simulink model "single_phase_full_bridge_inverter"  (R2021a)
settings: Solver=ode23tb  StartTime=0.0  StopTime=2*t  MaxStep=1e-4  RelTol=1e-3
values from neighbouring files (symbols this model uses):
  Ac = 1    [Inverter_parameters.m]
  Ar = ma*Ac    (= 0.5)    [Inverter_parameters.m]
  fc1 = mf1*f    (= 1000)    [Inverter_parameters.m]
  fc2 = mf2*f    (= 1150)    [Inverter_parameters.m]
  fr = 2*pi*f    (= 314.159265359)    [Inverter_parameters.m]
  L = X/(2*pi*f)    (= 0.0999493042617)    [Inverter_parameters.m]
  R = 100    [Inverter_parameters.m]
  Vin = 780    [Inverter_parameters.m]
libraries: spsRMSLib x5, spsIGBTDiodeLib x4, simulink x4, spsCurrentMeasurementLib x2, spsSeriesRLCBranchLib x1, spsVoltageMeasurementLib x1, spsDCVoltageSourceLib x1, spspowerguiLib x1
settings Model: Creator=HossamAladdin  LastModifiedBy=HossamAladdin
settings DataIOCC: ReturnWorkspaceOutputs=off

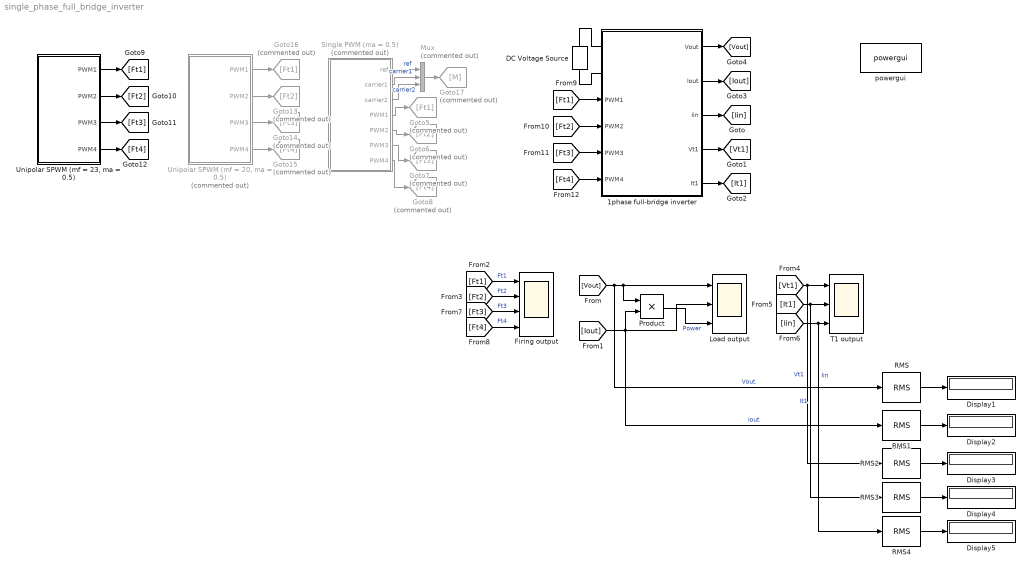
== system single_phase_full_bridge_inverter ==
  1phase full-bridge inverter : Subsystem
      settings: PortSchema="{\"entries\":[{\"content\":{\"sides\":[{\"content\":{\"connectorIds\":[\"LConn1\",\"LConn2\",\"In1\",\"In2\",\"In3\",\"In4\"]},\"type\":\"ConnectorPlacement.EquallySpacedRectSide\",\"uuid\":\"f4e4df3f-ffe1-4ba5-a3cb-8d734668f50c\"},{\"content\":{\"connectorIds\":[\"Out1\",\"Out2\",\"Out3\",\"Out4\",\"Out5\"],\"side\":\"RIGHT\"},\"type\":\"ConnectorPlacement.EquallySpacedRectSide\",\"uuid\":\"90fcdfa8-dce7-4e84-a242-f7f3ace87075\"},{\"content\":{\"connectorIds\":[],\"side\":\"TOP\"},\"type\":\"ConnectorPlacement.EquallySpacedRectSide\",\"uuid\":\"6c6a0c5d-cde1-4235-902c-253094bb6e2c\"}]},\"type\":\"ConnectorPlacement.EquallySpacedConnector\",\"uuid\":\"22214fd6-21aa-42b2-81ed-e947f83e4bbd\"}],\"packageUris\":[\"http://schema.mathworks.com/mf0/Connector/R2020b\"],\"version\":\"1.0\"}"
  DC Voltage Source : spsDCVoltageSourceLib/DC Voltage Source  Amplitude=Vin  Measurements=None
  Display{1..5} (5 alike) : Display
  Firing output : Scope  NumInputPorts=4
  Goto13 : Goto  Commented=on  GotoTag=Ft2
  Goto14 : Goto  Commented=on  GotoTag=Ft3
  Goto15 : Goto  Commented=on  GotoTag=Ft4
  Goto16 : Goto  Commented=on  GotoTag=Ft1
  Goto17 : Goto  Commented=on  GotoTag=M
  Goto5 : Goto  Commented=on  GotoTag=Ft1
  Goto6 : Goto  Commented=on  GotoTag=Ft2
  Goto7 : Goto  Commented=on  GotoTag=Ft3
  Goto8 : Goto  Commented=on  GotoTag=Ft4
  Load output : Scope  NumInputPorts=3
  Mux : Mux  Commented=on  Inputs=3
  Product : Product
  RMS{,1..4} (5 alike) : spsRMSLib/RMS  TrueRMS=on  Freq=50  RMSInit=0  Ts=0
  Single PWM (ma = 0.5) : Subsystem  Commented=on
  T1 output : Scope  NumInputPorts=3
  "Unipolar SPWM (mf = 20, ma = 0.5)" : Subsystem  Commented=on
  "Unipolar SPWM (mf = 23, ma = 0.5)" : Subsystem
  powergui : spspowerguiLib/powergui  Priority=1  SimulationMode=Discrete  SampleTime=1e-6  frequency=60  Iterations=50  frequencyindice=0  Pbase=100e6  ErrMax=1e-4  UnitsV=kV  UnitsW=MW  buscounter=0  FunctionMessages=off  echomessages=off  EnableUseOfTLC=off  CurrentSourceSwitches=off  DisableSnubberDevices=off  DisableRonSwitches=off  DisableVfSwitches=off  DisplayEquations=off  AutomaticDiscreteSolvers=off  SolverType=Tustin/Backward Euler (TBE)  Interpol=off  ExternalGateDelay=off  methode=off  Ts=100  x0status=blocks  SPID=on  SwTol=0  HookPort=off  NonlinearTolerance=1e-4  nMaxIteration=100  ContinueOnMaxIteration=off  RestoreLinks=warning  ResistiveCurrentMeasurement=off  Frange=[0:2:500]  Ylog=off  Xlog=on  ShowGrid=off  save=off  variable=ZData  structure=0  ZoomFFT=off  StartTime=0.0  cycles=1  DisplayStyle=1  fundamental=60  FreqAxis=off  MaxFrequency=1000  frequencyindicesteady=1  RmsSteady=1  display=off
  wires:
  1phase full-bridge inverter/5(It1) -> [It1]
  1phase full-bridge inverter/4(Vt1) -> [Vt1]
  1phase full-bridge inverter/2(Iout) -> [Iout]
  [Vt1] -> T1 output/1, RMS2/1  "Vt1"
  1phase full-bridge inverter/3(Iin) -> [Iin]
  1phase full-bridge inverter/1(Vout) -> [Vout]
  [Vout] -> RMS/1, Load output/1, Product/1  "Vout"
  [Ft2] -> Firing output/2  "Ft2"
  [Ft1] -> Firing output/1  "Ft1"
  [It1] -> T1 output/2, RMS3/1  "It1"
  [Iin] -> RMS4/1, T1 output/3  "Iin"
  [Iout] -> RMS1/1, Product/2, Load output/2  "Iout"
  Product/1 -> Load output/3  "Power"
  Single PWM (ma = 0.5)/4(PWM1) -> Goto5/1
  Single PWM (ma = 0.5)/5(PWM2) -> Goto6/1
  "Unipolar SPWM (mf = 23, ma = 0.5)"/4(PWM4) -> [Ft4]
  "Unipolar SPWM (mf = 23, ma = 0.5)"/1(PWM1) -> [Ft1]
  "Unipolar SPWM (mf = 20, ma = 0.5)"/1(PWM1) -> Goto16/1
  "Unipolar SPWM (mf = 20, ma = 0.5)"/4(PWM4) -> Goto15/1
  [Ft3] -> Firing output/3  "Ft3"
  [Ft4] -> Firing output/4  "Ft4"
  "Unipolar SPWM (mf = 20, ma = 0.5)"/2(PWM2) -> Goto13/1
  "Unipolar SPWM (mf = 20, ma = 0.5)"/3(PWM3) -> Goto14/1
  Single PWM (ma = 0.5)/7(PWM4) -> Goto8/1
  Single PWM (ma = 0.5)/6(PWM3) -> Goto7/1
  "Unipolar SPWM (mf = 23, ma = 0.5)"/2(PWM2) -> [Ft2]
  "Unipolar SPWM (mf = 23, ma = 0.5)"/3(PWM3) -> [Ft3]
  [Ft1] -> 1phase full-bridge inverter/1(PWM1)
  [Ft2] -> 1phase full-bridge inverter/2(PWM2)
  [Ft3] -> 1phase full-bridge inverter/3(PWM3)
  [Ft4] -> 1phase full-bridge inverter/4(PWM4)
  Single PWM (ma = 0.5)/1(ref) -> Mux/1  "ref"
  Single PWM (ma = 0.5)/2(carrier1) -> Mux/2  "carrier1"
  Single PWM (ma = 0.5)/3(carrier2) -> Mux/3  "carrier2"
  Mux/1 -> Goto17/1
  RMS4/1 -> Display5/1
  RMS1/1 -> Display2/1
  RMS3/1 -> Display4/1
  RMS2/1 -> Display3/1
  RMS/1 -> Display1/1
  connections:
  1phase full-bridge inverter/LConn1 -- DC Voltage Source/RConn1
  1phase full-bridge inverter/LConn2 -- DC Voltage Source/LConn1

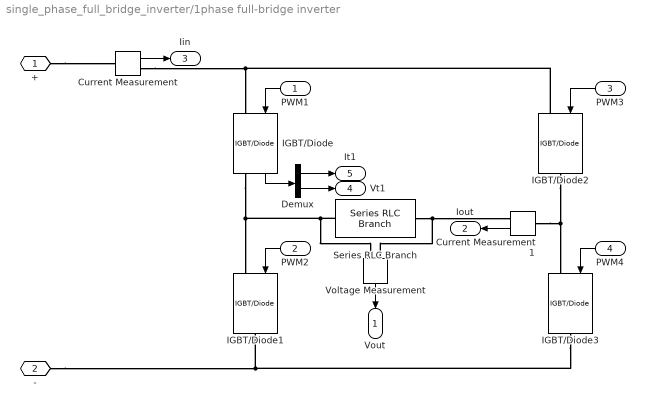
== system single_phase_full_bridge_inverter/1phase full-bridge inverter ==
  PWM1 : Inport
  PWM2 : Inport  Port=2
  PWM3 : Inport  Port=3
  PWM4 : Inport  Port=4
  Current Measurement : spsCurrentMeasurementLib/Current Measurement  PhasorSimulation=off  OutputType=Complex  PSBequivalent=0
  Current Measurement1 : spsCurrentMeasurementLib/Current Measurement  PhasorSimulation=off  OutputType=Complex  PSBequivalent=0
  Demux : Demux  Outputs=2
  IGBT/Diode : spsIGBTDiodeLib/IGBT//Diode  Ron=1e-3  Rs=1e5  Cs=inf  Measurements=on
  IGBT/Diode1 : spsIGBTDiodeLib/IGBT//Diode  Ron=1e-3  Rs=1e5  Cs=inf  Measurements=off
  IGBT/Diode2 : spsIGBTDiodeLib/IGBT//Diode  Ron=1e-3  Rs=1e5  Cs=inf  Measurements=off
  IGBT/Diode3 : spsIGBTDiodeLib/IGBT//Diode  Ron=1e-3  Rs=1e5  Cs=inf  Measurements=off
  Series RLC Branch : spsSeriesRLCBranchLib/Series RLC Branch  LConnTagsString=__new0  RConnTagsString=__new0  BranchType=RL  Resistance=R  Inductance=L  SetiL0=off  InitialCurrent=0  Capacitance=1e-6  Setx0=off  InitialVoltage=0  Measurements=None
  Voltage Measurement : spsVoltageMeasurementLib/Voltage Measurement  PhasorSimulation=off  OutputType=Complex  PSBequivalent=0
  + : PMIOPort  Side=Left
  - : PMIOPort  Port=2  Side=Left
  Vout : Outport
  Iout : Outport  Port=2
  Iin : Outport  Port=3
  Vt1 : Outport  Port=4
  It1 : Outport  Port=5
  wires:
  PWM1/1 -> IGBT/Diode/1
  Current Measurement/1 -> Iin/1
  Voltage Measurement/1 -> Vout/1
  Current Measurement1/1 -> Iout/1
  PWM3/1 -> IGBT/Diode2/1
  PWM2/1 -> IGBT/Diode1/1
  PWM4/1 -> IGBT/Diode3/1
  IGBT/Diode/1 -> Demux/1
  Demux/1 -> It1/1
  Demux/2 -> Vt1/1
  connections:
  Series RLC Branch/RConn1 -- Voltage Measurement/LConn2 -- Current Measurement1/RConn1
  Current Measurement1/LConn1 -- IGBT/Diode2/RConn1 -- IGBT/Diode3/LConn1
  IGBT/Diode2/LConn1 -- IGBT/Diode/LConn1 -- Current Measurement/RConn1
  +/RConn1 -- Current Measurement/LConn1
  IGBT/Diode3/RConn1 -- -/RConn1 -- IGBT/Diode1/RConn1
  Series RLC Branch/LConn1 -- IGBT/Diode/RConn1 -- IGBT/Diode1/LConn1 -- Voltage Measurement/LConn1

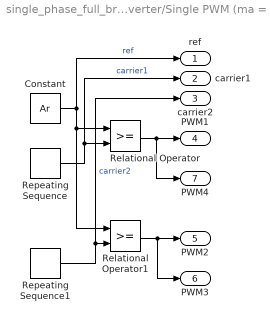
== system single_phase_full_bridge_inverter/Single PWM (ma = 0.5) ==
  Constant : Constant  Value=Ar
  Relational Operator : RelationalOperator  OutDataTypeStr=boolean  RndMeth=Simplest
  Relational Operator1 : RelationalOperator  OutDataTypeStr=boolean  RndMeth=Simplest
  Repeating Sequence : simulink/Sources/Repeating Sequence  rep_seq_t=[0 t/4 t/2 0.01001 t]  rep_seq_y=[Ac 0 Ac 1.001 1.001]
  Repeating Sequence1 : simulink/Sources/Repeating Sequence  rep_seq_t=[0 t/2 0.01001 3*t/4 t]  rep_seq_y=[1.001 1.001 Ac 0 Ac]
  ref : Outport
  carrier1 : Outport  Port=2
  carrier2 : Outport  Port=3
  PWM1 : Outport  Port=4
  PWM2 : Outport  Port=5
  PWM3 : Outport  Port=6
  PWM4 : Outport  Port=7
  wires:
  Relational Operator1/1 -> PWM3/1, PWM2/1
  Repeating Sequence/1 -> carrier1/1, Relational Operator/2  "carrier1"
  Repeating Sequence1/1 -> carrier2/1, Relational Operator1/2  "carrier2"
  Constant/1 -> ref/1, Relational Operator/1, Relational Operator1/1  "ref"
  Relational Operator/1 -> PWM4/1, PWM1/1

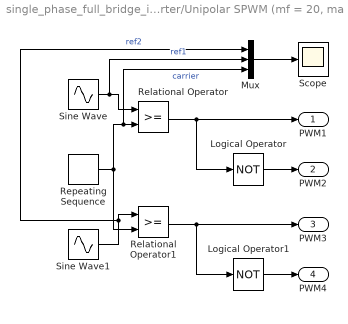
== system single_phase_full_bridge_inverter/Unipolar SPWM (mf = 20, ma = 0.5) ==
  Logical Operator : Logic  Operator=NOT  AllPortsSameDT=off  OutDataTypeStr=boolean
  Logical Operator1 : Logic  Operator=NOT  AllPortsSameDT=off  OutDataTypeStr=boolean
  Mux : Mux  Inputs=3
  Relational Operator : RelationalOperator  OutDataTypeStr=boolean  RndMeth=Simplest
  Relational Operator1 : RelationalOperator  OutDataTypeStr=boolean  RndMeth=Simplest
  Repeating Sequence : simulink/Sources/Repeating Sequence  rep_seq_t=[0 (1/fc1)/4 (1/fc1)/2 (3/fc1)/4 (1/fc1)]  rep_seq_y=[0 Ac 0 -Ac 0]
  Scope : Scope
  Sine Wave : Sin  Amplitude=Ar  Frequency=fr  SampleTime=0
  Sine Wave1 : Sin  Amplitude=Ar  Frequency=fr  Phase=pi  SampleTime=0
  PWM1 : Outport
  PWM2 : Outport  Port=2
  PWM3 : Outport  Port=3
  PWM4 : Outport  Port=4
  wires:
  Relational Operator/1 -> PWM1/1, Logical Operator/1
  Logical Operator1/1 -> PWM4/1
  Repeating Sequence/1 -> Relational Operator1/2, Mux/3, Relational Operator/2  "carrier"
  Sine Wave/1 -> Mux/2, Relational Operator/1  "ref1"
  Logical Operator/1 -> PWM2/1
  Sine Wave1/1 -> Relational Operator1/1, Mux/1  "ref2"
  Relational Operator1/1 -> Logical Operator1/1, PWM3/1
  Mux/1 -> Scope/1

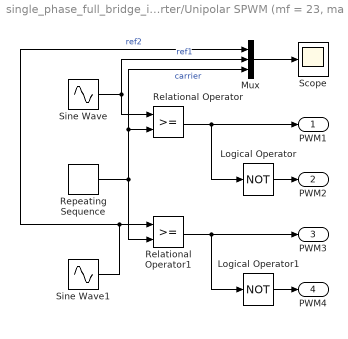
== system single_phase_full_bridge_inverter/Unipolar SPWM (mf = 23, ma = 0.5) ==
  Logical Operator : Logic  Operator=NOT  AllPortsSameDT=off  OutDataTypeStr=boolean
  Logical Operator1 : Logic  Operator=NOT  AllPortsSameDT=off  OutDataTypeStr=boolean
  Mux : Mux  Inputs=3
  Relational Operator : RelationalOperator  OutDataTypeStr=boolean  RndMeth=Simplest
  Relational Operator1 : RelationalOperator  OutDataTypeStr=boolean  RndMeth=Simplest
  Repeating Sequence : simulink/Sources/Repeating Sequence  rep_seq_t=[0 (1/fc2)/4 (1/fc2)/2 (3/fc2)/4 (1/fc2)]  rep_seq_y=[0 Ac 0 -Ac 0]
  Scope : Scope
  Sine Wave : Sin  Amplitude=Ar  Frequency=fr  SampleTime=0
  Sine Wave1 : Sin  Amplitude=Ar  Frequency=fr  Phase=pi  SampleTime=0
  PWM1 : Outport
  PWM2 : Outport  Port=2
  PWM3 : Outport  Port=3
  PWM4 : Outport  Port=4
  wires:
  Relational Operator/1 -> PWM1/1, Logical Operator/1
  Relational Operator1/1 -> Logical Operator1/1, PWM3/1
  Logical Operator/1 -> PWM2/1
  Logical Operator1/1 -> PWM4/1
  Repeating Sequence/1 -> Mux/3, Relational Operator/2, Relational Operator1/2  "carrier"
  Sine Wave/1 -> Mux/2, Relational Operator/1  "ref1"
  Mux/1 -> Scope/1
  Sine Wave1/1 -> Relational Operator1/1, Mux/1  "ref2"
